simulink model "uwb_hw_cosim_kintex"  (Simulink 8.0)
settings: Solver=ode45  StartTime=0.0  StopTime=33  RelTol=1e-3
InitFcn:
  | clear
  | %set_channel;
  | load channel;
  | Int_Data_input;
StopFcn:
  | bit_to_dec_excel;
  | abc=1;
values from neighbouring files (symbols this model uses):
  bit_rate = 9.7656e5    (= 976560)    [Int_Data_input.m]
undefined symbols (not defined in the file or in its folder): rsgenpoly
libraries: commutil2 x88, simulink x53, dspmtrx3 x32, dspindex x16, commcnvcod2 x8, commblkcod2 x8, dspsigops x3, commsink2 x2, xbsIndex_r4 x1, commchan3 x1, JTAGRuntimeCosim_r4 x1
(part 4 of 5)

== system uwb_hw_cosim_kintex/Subsystem2/Transmit2/Spreading/Hop10/Subsystem5 ==
  In1 : Inport
  matrix : Inport  Port=2
  CONST3 : Constant  Value=zeros(1,320)  VectorParams1D=off  OutDataTypeStr=int8  SampleTime=1
      settings: SamplingMode=Frame based
  Compare To Zero : simulink/Logic and Bit Operations/Compare To Zero  relop=>  OutDataTypeStr=uint8  ZeroCross=off
  Enabled Subsystem : Subsystem  TreatAsAtomicUnit=on
  Enabled Subsystem1 : Subsystem  TreatAsAtomicUnit=on
  Logical Operator : Logic  Operator=NOT  AllPortsSameDT=off  OutDataTypeStr=boolean
  Merge : Merge
  Reshape2 : Reshape  OutputDimensionality=Column vector (2-D)  OutputDimensions=[10,1]
  Out1 : Outport
  wires:
  CONST3/1 -> Reshape2/1
  Logical Operator/1 -> Enabled Subsystem/Enable
  Enabled Subsystem/1(Out1) -> Merge/2
  Enabled Subsystem1/1(Out1) -> Merge/1
  Compare To Zero/1 -> Enabled Subsystem1/Enable, Logical Operator/1
  Reshape2/1 -> Enabled Subsystem1/1(In1)
  matrix/1 -> Enabled Subsystem/1(In1)
  In1/1 -> Compare To Zero/1
  Merge/1 -> Out1/1

== system uwb_hw_cosim_kintex/Subsystem2/Transmit2/Spreading/Hop11/Kron ==
  p : Inport
  -p : Inport  Port=2
  sel : Inport  Port=3
  Compare To Zero : simulink/Logic and Bit Operations/Compare To Zero  relop=>  OutDataTypeStr=uint8  ZeroCross=off
  Enabled Subsystem : Subsystem  TreatAsAtomicUnit=on
  Enabled Subsystem1 : Subsystem  TreatAsAtomicUnit=on
  Logical Operator : Logic  Operator=NOT  AllPortsSameDT=off  OutDataTypeStr=boolean
  Merge : Merge
  burst : Outport
  wires:
  Logical Operator/1 -> Enabled Subsystem/Enable
  Compare To Zero/1 -> Enabled Subsystem1/Enable, Logical Operator/1
  sel/1 -> Compare To Zero/1
  -p/1 -> Enabled Subsystem/1(In1)
  Enabled Subsystem/1(Out1) -> Merge/2
  Enabled Subsystem1/1(Out1) -> Merge/1
  p/1 -> Enabled Subsystem1/1(In1)
  Merge/1 -> burst/1

== system uwb_hw_cosim_kintex/Subsystem2/Transmit2/Spreading/Hop11/Kron1 ==
  p : Inport
  -p : Inport  Port=2
  sel : Inport  Port=3
  Compare To Zero : simulink/Logic and Bit Operations/Compare To Zero  relop=>  OutDataTypeStr=uint8  ZeroCross=off
  Enabled Subsystem : Subsystem  TreatAsAtomicUnit=on
  Enabled Subsystem1 : Subsystem  TreatAsAtomicUnit=on
  Logical Operator : Logic  Operator=NOT  AllPortsSameDT=off  OutDataTypeStr=boolean
  Merge : Merge
  burst : Outport
  wires:
  Merge/1 -> burst/1
  p/1 -> Enabled Subsystem1/1(In1)
  Enabled Subsystem1/1(Out1) -> Merge/1
  Enabled Subsystem/1(Out1) -> Merge/2
  -p/1 -> Enabled Subsystem/1(In1)
  sel/1 -> Compare To Zero/1
  Compare To Zero/1 -> Logical Operator/1, Enabled Subsystem1/Enable
  Logical Operator/1 -> Enabled Subsystem/Enable

== system uwb_hw_cosim_kintex/Subsystem2/Transmit2/Spreading/Hop11/Subsystem2 ==
  note: 16bit cua S mã hóa 1 cum xung gause 320 diem, them 7x320 diem 0
      | de tao ra 1/2 frame chua tin hieu
  In1 : Inport
  Buffer 48bit1 : Buffer  N=16
  Frame Conversion1 : FrameConversion
  Reshape3 : Reshape  OutputDimensionality=Customize  OutputDimensions=[320,1]
  Transpose1 : dspmtrx3/Transpose  Hermitian=off  overflowFlag=off
  Out1 : Outport
  wires:
  Frame Conversion1/1 -> Out1/1
  In1/1 -> Buffer 48bit1/1
  Reshape3/1 -> Frame Conversion1/1
  Transpose1/1 -> Reshape3/1
  Buffer 48bit1/1 -> Transpose1/1

== system uwb_hw_cosim_kintex/Subsystem2/Transmit2/Spreading/Hop11/Subsystem3 ==
  In1 : Inport
  Add1 : Sum  Inputs=+-
  Bi2De2 : commutil2/Bit to Integer Converter  nbits=2  bitOrder=MSB first  signedOutputValues=Unsigned  outDtype=int8  outDtypeSigned=Inherit via internal rule
  Gain2 : Gain  Gain=0.5  OutDataTypeStr=int8  RndMeth=Zero
  Gain4 : Gain  Gain=2  OutDataTypeStr=int8
  position : Outport
  sign : Outport  Port=2
  wires:
  Add1/1 -> position/1
  Bi2De2/1 -> Gain2/1, Add1/1
  Gain4/1 -> Add1/2
  Gain2/1 -> sign/1, Gain4/1
  In1/1 -> Bi2De2/1

== system uwb_hw_cosim_kintex/Subsystem2/Transmit2/Spreading/Hop11/Subsystem5 ==
  In1 : Inport
  matrix : Inport  Port=2
  CONST3 : Constant  Value=zeros(1,320)  VectorParams1D=off  OutDataTypeStr=int8  SampleTime=1
      settings: SamplingMode=Frame based
  Compare To Zero : simulink/Logic and Bit Operations/Compare To Zero  relop=>  OutDataTypeStr=uint8  ZeroCross=off
  Enabled Subsystem : Subsystem  TreatAsAtomicUnit=on
  Enabled Subsystem1 : Subsystem  TreatAsAtomicUnit=on
  Logical Operator : Logic  Operator=NOT  AllPortsSameDT=off  OutDataTypeStr=boolean
  Merge : Merge
  Reshape2 : Reshape  OutputDimensionality=Column vector (2-D)  OutputDimensions=[10,1]
  Out1 : Outport
  wires:
  Merge/1 -> Out1/1
  In1/1 -> Compare To Zero/1
  matrix/1 -> Enabled Subsystem/1(In1)
  Reshape2/1 -> Enabled Subsystem1/1(In1)
  Compare To Zero/1 -> Logical Operator/1, Enabled Subsystem1/Enable
  Enabled Subsystem1/1(Out1) -> Merge/1
  Enabled Subsystem/1(Out1) -> Merge/2
  Logical Operator/1 -> Enabled Subsystem/Enable
  CONST3/1 -> Reshape2/1

== system uwb_hw_cosim_kintex/Subsystem2/Transmit2/Spreading/Hop12/Kron ==
  p : Inport
  -p : Inport  Port=2
  sel : Inport  Port=3
  Compare To Zero : simulink/Logic and Bit Operations/Compare To Zero  relop=>  OutDataTypeStr=uint8  ZeroCross=off
  Enabled Subsystem : Subsystem  TreatAsAtomicUnit=on
  Enabled Subsystem1 : Subsystem  TreatAsAtomicUnit=on
  Logical Operator : Logic  Operator=NOT  AllPortsSameDT=off  OutDataTypeStr=boolean
  Merge : Merge
  burst : Outport
  wires:
  Logical Operator/1 -> Enabled Subsystem/Enable
  Compare To Zero/1 -> Enabled Subsystem1/Enable, Logical Operator/1
  sel/1 -> Compare To Zero/1
  -p/1 -> Enabled Subsystem/1(In1)
  Enabled Subsystem/1(Out1) -> Merge/2
  Enabled Subsystem1/1(Out1) -> Merge/1
  p/1 -> Enabled Subsystem1/1(In1)
  Merge/1 -> burst/1

== system uwb_hw_cosim_kintex/Subsystem2/Transmit2/Spreading/Hop12/Kron1 ==
  p : Inport
  -p : Inport  Port=2
  sel : Inport  Port=3
  Compare To Zero : simulink/Logic and Bit Operations/Compare To Zero  relop=>  OutDataTypeStr=uint8  ZeroCross=off
  Enabled Subsystem : Subsystem  TreatAsAtomicUnit=on
  Enabled Subsystem1 : Subsystem  TreatAsAtomicUnit=on
  Logical Operator : Logic  Operator=NOT  AllPortsSameDT=off  OutDataTypeStr=boolean
  Merge : Merge
  burst : Outport
  wires:
  Merge/1 -> burst/1
  p/1 -> Enabled Subsystem1/1(In1)
  Enabled Subsystem1/1(Out1) -> Merge/1
  Enabled Subsystem/1(Out1) -> Merge/2
  -p/1 -> Enabled Subsystem/1(In1)
  sel/1 -> Compare To Zero/1
  Compare To Zero/1 -> Logical Operator/1, Enabled Subsystem1/Enable
  Logical Operator/1 -> Enabled Subsystem/Enable

== system uwb_hw_cosim_kintex/Subsystem2/Transmit2/Spreading/Hop12/Subsystem2 ==
  note: 16bit cua S mã hóa 1 cum xung gause 320 diem, them 7x320 diem 0
      | de tao ra 1/2 frame chua tin hieu
  In1 : Inport
  Buffer 48bit1 : Buffer  N=16
  Frame Conversion1 : FrameConversion
  Reshape3 : Reshape  OutputDimensionality=Customize  OutputDimensions=[320,1]
  Transpose1 : dspmtrx3/Transpose  Hermitian=off  overflowFlag=off
  Out1 : Outport
  wires:
  Frame Conversion1/1 -> Out1/1
  In1/1 -> Buffer 48bit1/1
  Reshape3/1 -> Frame Conversion1/1
  Transpose1/1 -> Reshape3/1
  Buffer 48bit1/1 -> Transpose1/1

== system uwb_hw_cosim_kintex/Subsystem2/Transmit2/Spreading/Hop12/Subsystem3 ==
  In1 : Inport
  Add1 : Sum  Inputs=+-
  Bi2De2 : commutil2/Bit to Integer Converter  nbits=2  bitOrder=MSB first  signedOutputValues=Unsigned  outDtype=int8  outDtypeSigned=Inherit via internal rule
  Gain2 : Gain  Gain=0.5  OutDataTypeStr=int8  RndMeth=Zero
  Gain4 : Gain  Gain=2  OutDataTypeStr=int8
  position : Outport
  sign : Outport  Port=2
  wires:
  Add1/1 -> position/1
  Bi2De2/1 -> Gain2/1, Add1/1
  Gain4/1 -> Add1/2
  Gain2/1 -> sign/1, Gain4/1
  In1/1 -> Bi2De2/1

== system uwb_hw_cosim_kintex/Subsystem2/Transmit2/Spreading/Hop12/Subsystem5 ==
  In1 : Inport
  matrix : Inport  Port=2
  CONST3 : Constant  Value=zeros(1,320)  VectorParams1D=off  OutDataTypeStr=int8  SampleTime=1
      settings: SamplingMode=Frame based
  Compare To Zero : simulink/Logic and Bit Operations/Compare To Zero  relop===  OutDataTypeStr=uint8  ZeroCross=off
  Enabled Subsystem : Subsystem  TreatAsAtomicUnit=on
  Enabled Subsystem1 : Subsystem  TreatAsAtomicUnit=on
  Logical Operator : Logic  Operator=NOT  AllPortsSameDT=off  OutDataTypeStr=boolean
  Merge : Merge
  Reshape2 : Reshape  OutputDimensionality=Column vector (2-D)  OutputDimensions=[10,1]
  Out1 : Outport
  wires:
  Merge/1 -> Out1/1
  In1/1 -> Compare To Zero/1
  Reshape2/1 -> Enabled Subsystem1/1(In1)
  Compare To Zero/1 -> Logical Operator/1, Enabled Subsystem1/Enable
  Enabled Subsystem1/1(Out1) -> Merge/1
  Enabled Subsystem/1(Out1) -> Merge/2
  Logical Operator/1 -> Enabled Subsystem/Enable
  CONST3/1 -> Reshape2/1
  matrix/1 -> Enabled Subsystem/1(In1)

== system uwb_hw_cosim_kintex/Subsystem2/Transmit2/Spreading/Hop13/Kron ==
  p : Inport
  -p : Inport  Port=2
  sel : Inport  Port=3
  Compare To Zero : simulink/Logic and Bit Operations/Compare To Zero  relop=>  OutDataTypeStr=uint8  ZeroCross=off
  Enabled Subsystem : Subsystem  TreatAsAtomicUnit=on
  Enabled Subsystem1 : Subsystem  TreatAsAtomicUnit=on
  Logical Operator : Logic  Operator=NOT  AllPortsSameDT=off  OutDataTypeStr=boolean
  Merge : Merge
  burst : Outport
  wires:
  Merge/1 -> burst/1
  p/1 -> Enabled Subsystem1/1(In1)
  Enabled Subsystem1/1(Out1) -> Merge/1
  Enabled Subsystem/1(Out1) -> Merge/2
  -p/1 -> Enabled Subsystem/1(In1)
  sel/1 -> Compare To Zero/1
  Compare To Zero/1 -> Logical Operator/1, Enabled Subsystem1/Enable
  Logical Operator/1 -> Enabled Subsystem/Enable

== system uwb_hw_cosim_kintex/Subsystem2/Transmit2/Spreading/Hop13/Kron1 ==
  p : Inport
  -p : Inport  Port=2
  sel : Inport  Port=3
  Compare To Zero : simulink/Logic and Bit Operations/Compare To Zero  relop=>  OutDataTypeStr=uint8  ZeroCross=off
  Enabled Subsystem : Subsystem  TreatAsAtomicUnit=on
  Enabled Subsystem1 : Subsystem  TreatAsAtomicUnit=on
  Logical Operator : Logic  Operator=NOT  AllPortsSameDT=off  OutDataTypeStr=boolean
  Merge : Merge
  burst : Outport
  wires:
  Logical Operator/1 -> Enabled Subsystem/Enable
  Compare To Zero/1 -> Enabled Subsystem1/Enable, Logical Operator/1
  sel/1 -> Compare To Zero/1
  -p/1 -> Enabled Subsystem/1(In1)
  Enabled Subsystem/1(Out1) -> Merge/2
  Enabled Subsystem1/1(Out1) -> Merge/1
  p/1 -> Enabled Subsystem1/1(In1)
  Merge/1 -> burst/1

== system uwb_hw_cosim_kintex/Subsystem2/Transmit2/Spreading/Hop13/Subsystem2 ==
  note: 16bit cua S mã hóa 1 cum xung gause 320 diem, them 7x320 diem 0
      | de tao ra 1/2 frame chua tin hieu
  In1 : Inport
  Buffer 48bit1 : Buffer  N=16
  Frame Conversion1 : FrameConversion
  Reshape3 : Reshape  OutputDimensionality=Customize  OutputDimensions=[320,1]
  Transpose1 : dspmtrx3/Transpose  Hermitian=off  overflowFlag=off
  Out1 : Outport
  wires:
  Buffer 48bit1/1 -> Transpose1/1
  Transpose1/1 -> Reshape3/1
  Reshape3/1 -> Frame Conversion1/1
  In1/1 -> Buffer 48bit1/1
  Frame Conversion1/1 -> Out1/1

== system uwb_hw_cosim_kintex/Subsystem2/Transmit2/Spreading/Hop13/Subsystem3 ==
  In1 : Inport
  Add1 : Sum  Inputs=+-
  Bi2De2 : commutil2/Bit to Integer Converter  nbits=2  bitOrder=MSB first  signedOutputValues=Unsigned  outDtype=int8  outDtypeSigned=Inherit via internal rule
  Gain2 : Gain  Gain=0.5  OutDataTypeStr=int8  RndMeth=Zero
  Gain4 : Gain  Gain=2  OutDataTypeStr=int8
  position : Outport
  sign : Outport  Port=2
  wires:
  In1/1 -> Bi2De2/1
  Gain2/1 -> Gain4/1, sign/1
  Gain4/1 -> Add1/2
  Bi2De2/1 -> Add1/1, Gain2/1
  Add1/1 -> position/1

== system uwb_hw_cosim_kintex/Subsystem2/Transmit2/Spreading/Hop13/Subsystem5 ==
  In1 : Inport
  matrix : Inport  Port=2
  CONST3 : Constant  Value=zeros(1,320)  VectorParams1D=off  OutDataTypeStr=int8  SampleTime=1
      settings: SamplingMode=Frame based
  Compare To Zero : simulink/Logic and Bit Operations/Compare To Zero  relop===  OutDataTypeStr=uint8  ZeroCross=off
  Enabled Subsystem : Subsystem  TreatAsAtomicUnit=on
  Enabled Subsystem1 : Subsystem  TreatAsAtomicUnit=on
  Logical Operator : Logic  Operator=NOT  AllPortsSameDT=off  OutDataTypeStr=boolean
  Merge : Merge
  Reshape2 : Reshape  OutputDimensionality=Column vector (2-D)  OutputDimensions=[10,1]
  Out1 : Outport
  wires:
  matrix/1 -> Enabled Subsystem/1(In1)
  CONST3/1 -> Reshape2/1
  Logical Operator/1 -> Enabled Subsystem/Enable
  Enabled Subsystem/1(Out1) -> Merge/2
  Enabled Subsystem1/1(Out1) -> Merge/1
  Compare To Zero/1 -> Enabled Subsystem1/Enable, Logical Operator/1
  Reshape2/1 -> Enabled Subsystem1/1(In1)
  In1/1 -> Compare To Zero/1
  Merge/1 -> Out1/1

== system uwb_hw_cosim_kintex/Subsystem2/Transmit2/Spreading/Hop14/Kron ==
  p : Inport
  -p : Inport  Port=2
  sel : Inport  Port=3
  Compare To Zero : simulink/Logic and Bit Operations/Compare To Zero  relop=>  OutDataTypeStr=uint8  ZeroCross=off
  Enabled Subsystem : Subsystem  TreatAsAtomicUnit=on
  Enabled Subsystem1 : Subsystem  TreatAsAtomicUnit=on
  Logical Operator : Logic  Operator=NOT  AllPortsSameDT=off  OutDataTypeStr=boolean
  Merge : Merge
  burst : Outport
  wires:
  Logical Operator/1 -> Enabled Subsystem/Enable
  Compare To Zero/1 -> Enabled Subsystem1/Enable, Logical Operator/1
  sel/1 -> Compare To Zero/1
  -p/1 -> Enabled Subsystem/1(In1)
  Enabled Subsystem/1(Out1) -> Merge/2
  Enabled Subsystem1/1(Out1) -> Merge/1
  p/1 -> Enabled Subsystem1/1(In1)
  Merge/1 -> burst/1

== system uwb_hw_cosim_kintex/Subsystem2/Transmit2/Spreading/Hop14/Kron1 ==
  p : Inport
  -p : Inport  Port=2
  sel : Inport  Port=3
  Compare To Zero : simulink/Logic and Bit Operations/Compare To Zero  relop=>  OutDataTypeStr=uint8  ZeroCross=off
  Enabled Subsystem : Subsystem  TreatAsAtomicUnit=on
  Enabled Subsystem1 : Subsystem  TreatAsAtomicUnit=on
  Logical Operator : Logic  Operator=NOT  AllPortsSameDT=off  OutDataTypeStr=boolean
  Merge : Merge
  burst : Outport
  wires:
  Merge/1 -> burst/1
  p/1 -> Enabled Subsystem1/1(In1)
  Enabled Subsystem1/1(Out1) -> Merge/1
  Enabled Subsystem/1(Out1) -> Merge/2
  -p/1 -> Enabled Subsystem/1(In1)
  sel/1 -> Compare To Zero/1
  Compare To Zero/1 -> Logical Operator/1, Enabled Subsystem1/Enable
  Logical Operator/1 -> Enabled Subsystem/Enable

== system uwb_hw_cosim_kintex/Subsystem2/Transmit2/Spreading/Hop14/Subsystem2 ==
  note: 16bit cua S mã hóa 1 cum xung gause 320 diem, them 7x320 diem 0
      | de tao ra 1/2 frame chua tin hieu
  In1 : Inport
  Buffer 48bit1 : Buffer  N=16
  Frame Conversion1 : FrameConversion
  Reshape3 : Reshape  OutputDimensionality=Customize  OutputDimensions=[320,1]
  Transpose1 : dspmtrx3/Transpose  Hermitian=off  overflowFlag=off
  Out1 : Outport
  wires:
  Frame Conversion1/1 -> Out1/1
  In1/1 -> Buffer 48bit1/1
  Reshape3/1 -> Frame Conversion1/1
  Transpose1/1 -> Reshape3/1
  Buffer 48bit1/1 -> Transpose1/1

== system uwb_hw_cosim_kintex/Subsystem2/Transmit2/Spreading/Hop14/Subsystem3 ==
  In1 : Inport
  Add1 : Sum  Inputs=+-
  Bi2De2 : commutil2/Bit to Integer Converter  nbits=2  bitOrder=MSB first  signedOutputValues=Unsigned  outDtype=int8  outDtypeSigned=Inherit via internal rule
  Gain2 : Gain  Gain=0.5  OutDataTypeStr=int8  RndMeth=Zero
  Gain4 : Gain  Gain=2  OutDataTypeStr=int8
  position : Outport
  sign : Outport  Port=2
  wires:
  Add1/1 -> position/1
  Bi2De2/1 -> Gain2/1, Add1/1
  Gain4/1 -> Add1/2
  Gain2/1 -> sign/1, Gain4/1
  In1/1 -> Bi2De2/1

== system uwb_hw_cosim_kintex/Subsystem2/Transmit2/Spreading/Hop14/Subsystem5 ==
  In1 : Inport
  matrix : Inport  Port=2
  CONST3 : Constant  Value=zeros(1,320)  VectorParams1D=off  OutDataTypeStr=int8  SampleTime=1
      settings: SamplingMode=Frame based
  Compare To Zero : simulink/Logic and Bit Operations/Compare To Zero  relop===  OutDataTypeStr=uint8  ZeroCross=off
  Enabled Subsystem : Subsystem  TreatAsAtomicUnit=on
  Enabled Subsystem1 : Subsystem  TreatAsAtomicUnit=on
  Logical Operator : Logic  Operator=NOT  AllPortsSameDT=off  OutDataTypeStr=boolean
  Merge : Merge
  Reshape2 : Reshape  OutputDimensionality=Column vector (2-D)  OutputDimensions=[10,1]
  Out1 : Outport
  wires:
  Merge/1 -> Out1/1
  In1/1 -> Compare To Zero/1
  Reshape2/1 -> Enabled Subsystem1/1(In1)
  Compare To Zero/1 -> Logical Operator/1, Enabled Subsystem1/Enable
  Enabled Subsystem1/1(Out1) -> Merge/1
  Enabled Subsystem/1(Out1) -> Merge/2
  Logical Operator/1 -> Enabled Subsystem/Enable
  CONST3/1 -> Reshape2/1
  matrix/1 -> Enabled Subsystem/1(In1)

== system uwb_hw_cosim_kintex/Subsystem2/Transmit2/Spreading/Hop15/Kron ==
  p : Inport
  -p : Inport  Port=2
  sel : Inport  Port=3
  Compare To Zero : simulink/Logic and Bit Operations/Compare To Zero  relop=>  OutDataTypeStr=uint8  ZeroCross=off
  Enabled Subsystem : Subsystem  TreatAsAtomicUnit=on
  Enabled Subsystem1 : Subsystem  TreatAsAtomicUnit=on
  Logical Operator : Logic  Operator=NOT  AllPortsSameDT=off  OutDataTypeStr=boolean
  Merge : Merge
  burst : Outport
  wires:
  Merge/1 -> burst/1
  p/1 -> Enabled Subsystem1/1(In1)
  Enabled Subsystem1/1(Out1) -> Merge/1
  Enabled Subsystem/1(Out1) -> Merge/2
  -p/1 -> Enabled Subsystem/1(In1)
  sel/1 -> Compare To Zero/1
  Compare To Zero/1 -> Logical Operator/1, Enabled Subsystem1/Enable
  Logical Operator/1 -> Enabled Subsystem/Enable

== system uwb_hw_cosim_kintex/Subsystem2/Transmit2/Spreading/Hop15/Kron1 ==
  p : Inport
  -p : Inport  Port=2
  sel : Inport  Port=3
  Compare To Zero : simulink/Logic and Bit Operations/Compare To Zero  relop=>  OutDataTypeStr=uint8  ZeroCross=off
  Enabled Subsystem : Subsystem  TreatAsAtomicUnit=on
  Enabled Subsystem1 : Subsystem  TreatAsAtomicUnit=on
  Logical Operator : Logic  Operator=NOT  AllPortsSameDT=off  OutDataTypeStr=boolean
  Merge : Merge
  burst : Outport
  wires:
  Logical Operator/1 -> Enabled Subsystem/Enable
  Compare To Zero/1 -> Enabled Subsystem1/Enable, Logical Operator/1
  sel/1 -> Compare To Zero/1
  -p/1 -> Enabled Subsystem/1(In1)
  Enabled Subsystem/1(Out1) -> Merge/2
  Enabled Subsystem1/1(Out1) -> Merge/1
  p/1 -> Enabled Subsystem1/1(In1)
  Merge/1 -> burst/1

== system uwb_hw_cosim_kintex/Subsystem2/Transmit2/Spreading/Hop15/Subsystem2 ==
  note: 16bit cua S mã hóa 1 cum xung gause 320 diem, them 7x320 diem 0
      | de tao ra 1/2 frame chua tin hieu
  In1 : Inport
  Buffer 48bit1 : Buffer  N=16
  Frame Conversion1 : FrameConversion
  Reshape3 : Reshape  OutputDimensionality=Customize  OutputDimensions=[320,1]
  Transpose1 : dspmtrx3/Transpose  Hermitian=off  overflowFlag=off
  Out1 : Outport
  wires:
  Buffer 48bit1/1 -> Transpose1/1
  Transpose1/1 -> Reshape3/1
  Reshape3/1 -> Frame Conversion1/1
  In1/1 -> Buffer 48bit1/1
  Frame Conversion1/1 -> Out1/1

== system uwb_hw_cosim_kintex/Subsystem2/Transmit2/Spreading/Hop15/Subsystem3 ==
  In1 : Inport
  Add1 : Sum  Inputs=+-
  Bi2De2 : commutil2/Bit to Integer Converter  nbits=2  bitOrder=MSB first  signedOutputValues=Unsigned  outDtype=int8  outDtypeSigned=Inherit via internal rule
  Gain2 : Gain  Gain=0.5  OutDataTypeStr=int8  RndMeth=Zero
  Gain4 : Gain  Gain=2  OutDataTypeStr=int8
  position : Outport
  sign : Outport  Port=2
  wires:
  In1/1 -> Bi2De2/1
  Gain2/1 -> Gain4/1, sign/1
  Gain4/1 -> Add1/2
  Bi2De2/1 -> Add1/1, Gain2/1
  Add1/1 -> position/1

== system uwb_hw_cosim_kintex/Subsystem2/Transmit2/Spreading/Hop15/Subsystem5 ==
  In1 : Inport
  matrix : Inport  Port=2
  CONST3 : Constant  Value=zeros(1,320)  VectorParams1D=off  OutDataTypeStr=int8  SampleTime=1
      settings: SamplingMode=Frame based
  Compare To Zero : simulink/Logic and Bit Operations/Compare To Zero  relop===  OutDataTypeStr=uint8  ZeroCross=off
  Enabled Subsystem : Subsystem  TreatAsAtomicUnit=on
  Enabled Subsystem1 : Subsystem  TreatAsAtomicUnit=on
  Logical Operator : Logic  Operator=NOT  AllPortsSameDT=off  OutDataTypeStr=boolean
  Merge : Merge
  Reshape2 : Reshape  OutputDimensionality=Column vector (2-D)  OutputDimensions=[10,1]
  Out1 : Outport
  wires:
  matrix/1 -> Enabled Subsystem/1(In1)
  CONST3/1 -> Reshape2/1
  Logical Operator/1 -> Enabled Subsystem/Enable
  Enabled Subsystem/1(Out1) -> Merge/2
  Enabled Subsystem1/1(Out1) -> Merge/1
  Compare To Zero/1 -> Enabled Subsystem1/Enable, Logical Operator/1
  Reshape2/1 -> Enabled Subsystem1/1(In1)
  In1/1 -> Compare To Zero/1
  Merge/1 -> Out1/1

== system uwb_hw_cosim_kintex/Subsystem2/Transmit2/Spreading/Hop17/Kron ==
  p : Inport
  -p : Inport  Port=2
  sel : Inport  Port=3
  Compare To Zero : simulink/Logic and Bit Operations/Compare To Zero  relop=>  OutDataTypeStr=uint8  ZeroCross=off
  Enabled Subsystem : Subsystem  TreatAsAtomicUnit=on
  Enabled Subsystem1 : Subsystem  TreatAsAtomicUnit=on
  Logical Operator : Logic  Operator=NOT  AllPortsSameDT=off  OutDataTypeStr=boolean
  Merge : Merge
  burst : Outport
  wires:
  Merge/1 -> burst/1
  p/1 -> Enabled Subsystem1/1(In1)
  Enabled Subsystem1/1(Out1) -> Merge/1
  Enabled Subsystem/1(Out1) -> Merge/2
  -p/1 -> Enabled Subsystem/1(In1)
  sel/1 -> Compare To Zero/1
  Compare To Zero/1 -> Logical Operator/1, Enabled Subsystem1/Enable
  Logical Operator/1 -> Enabled Subsystem/Enable

== system uwb_hw_cosim_kintex/Subsystem2/Transmit2/Spreading/Hop17/Kron1 ==
  p : Inport
  -p : Inport  Port=2
  sel : Inport  Port=3
  Compare To Zero : simulink/Logic and Bit Operations/Compare To Zero  relop=>  OutDataTypeStr=uint8  ZeroCross=off
  Enabled Subsystem : Subsystem  TreatAsAtomicUnit=on
  Enabled Subsystem1 : Subsystem  TreatAsAtomicUnit=on
  Logical Operator : Logic  Operator=NOT  AllPortsSameDT=off  OutDataTypeStr=boolean
  Merge : Merge
  burst : Outport
  wires:
  Logical Operator/1 -> Enabled Subsystem/Enable
  Compare To Zero/1 -> Enabled Subsystem1/Enable, Logical Operator/1
  sel/1 -> Compare To Zero/1
  -p/1 -> Enabled Subsystem/1(In1)
  Enabled Subsystem/1(Out1) -> Merge/2
  Enabled Subsystem1/1(Out1) -> Merge/1
  p/1 -> Enabled Subsystem1/1(In1)
  Merge/1 -> burst/1

== system uwb_hw_cosim_kintex/Subsystem2/Transmit2/Spreading/Hop17/Subsystem2 ==
  note: 16bit cua S mã hóa 1 cum xung gause 320 diem, them 7x320 diem 0
      | de tao ra 1/2 frame chua tin hieu
  In1 : Inport
  Buffer 48bit1 : Buffer  N=16
  Frame Conversion1 : FrameConversion
  Reshape3 : Reshape  OutputDimensionality=Customize  OutputDimensions=[320,1]
  Transpose1 : dspmtrx3/Transpose  Hermitian=off  overflowFlag=off
  Out1 : Outport
  wires:
  Buffer 48bit1/1 -> Transpose1/1
  Transpose1/1 -> Reshape3/1
  Reshape3/1 -> Frame Conversion1/1
  In1/1 -> Buffer 48bit1/1
  Frame Conversion1/1 -> Out1/1

== system uwb_hw_cosim_kintex/Subsystem2/Transmit2/Spreading/Hop17/Subsystem3 ==
  In1 : Inport
  Add1 : Sum  Inputs=+-
  Bi2De2 : commutil2/Bit to Integer Converter  nbits=2  bitOrder=MSB first  signedOutputValues=Unsigned  outDtype=int8  outDtypeSigned=Inherit via internal rule
  Gain2 : Gain  Gain=0.5  OutDataTypeStr=int8  RndMeth=Zero
  Gain4 : Gain  Gain=2  OutDataTypeStr=int8
  position : Outport
  sign : Outport  Port=2
  wires:
  In1/1 -> Bi2De2/1
  Gain2/1 -> Gain4/1, sign/1
  Gain4/1 -> Add1/2
  Bi2De2/1 -> Add1/1, Gain2/1
  Add1/1 -> position/1

== system uwb_hw_cosim_kintex/Subsystem2/Transmit2/Spreading/Hop17/Subsystem5 ==
  In1 : Inport
  matrix : Inport  Port=2
  CONST3 : Constant  Value=zeros(1,320)  VectorParams1D=off  OutDataTypeStr=int8  SampleTime=1
      settings: SamplingMode=Frame based
  Compare To Zero : simulink/Logic and Bit Operations/Compare To Zero  relop===  OutDataTypeStr=uint8  ZeroCross=off
  Enabled Subsystem : Subsystem  TreatAsAtomicUnit=on
  Enabled Subsystem1 : Subsystem  TreatAsAtomicUnit=on
  Logical Operator : Logic  Operator=NOT  AllPortsSameDT=off  OutDataTypeStr=boolean
  Merge : Merge
  Reshape2 : Reshape  OutputDimensionality=Column vector (2-D)  OutputDimensions=[10,1]
  Out1 : Outport
  wires:
  matrix/1 -> Enabled Subsystem/1(In1)
  CONST3/1 -> Reshape2/1
  Logical Operator/1 -> Enabled Subsystem/Enable
  Enabled Subsystem/1(Out1) -> Merge/2
  Enabled Subsystem1/1(Out1) -> Merge/1
  Compare To Zero/1 -> Enabled Subsystem1/Enable, Logical Operator/1
  Reshape2/1 -> Enabled Subsystem1/1(In1)
  In1/1 -> Compare To Zero/1
  Merge/1 -> Out1/1

== system uwb_hw_cosim_kintex/Subsystem2/Transmit2/Spreading/Hop2/Kron ==
  p : Inport
  -p : Inport  Port=2
  sel : Inport  Port=3
  Compare To Zero : simulink/Logic and Bit Operations/Compare To Zero  relop=>  OutDataTypeStr=uint8  ZeroCross=off
  Enabled Subsystem : Subsystem  TreatAsAtomicUnit=on
  Enabled Subsystem1 : Subsystem  TreatAsAtomicUnit=on
  Logical Operator : Logic  Operator=NOT  AllPortsSameDT=off  OutDataTypeStr=boolean
  Merge : Merge
  burst : Outport
  wires:
  Merge/1 -> burst/1
  p/1 -> Enabled Subsystem1/1(In1)
  Enabled Subsystem1/1(Out1) -> Merge/1
  Enabled Subsystem/1(Out1) -> Merge/2
  -p/1 -> Enabled Subsystem/1(In1)
  sel/1 -> Compare To Zero/1
  Compare To Zero/1 -> Logical Operator/1, Enabled Subsystem1/Enable
  Logical Operator/1 -> Enabled Subsystem/Enable

== system uwb_hw_cosim_kintex/Subsystem2/Transmit2/Spreading/Hop2/Kron1 ==
  p : Inport
  -p : Inport  Port=2
  sel : Inport  Port=3
  Compare To Zero : simulink/Logic and Bit Operations/Compare To Zero  relop=>  OutDataTypeStr=uint8  ZeroCross=off
  Enabled Subsystem : Subsystem  TreatAsAtomicUnit=on
  Enabled Subsystem1 : Subsystem  TreatAsAtomicUnit=on
  Logical Operator : Logic  Operator=NOT  AllPortsSameDT=off  OutDataTypeStr=boolean
  Merge : Merge
  burst : Outport
  wires:
  Logical Operator/1 -> Enabled Subsystem/Enable
  Compare To Zero/1 -> Enabled Subsystem1/Enable, Logical Operator/1
  sel/1 -> Compare To Zero/1
  -p/1 -> Enabled Subsystem/1(In1)
  Enabled Subsystem/1(Out1) -> Merge/2
  Enabled Subsystem1/1(Out1) -> Merge/1
  p/1 -> Enabled Subsystem1/1(In1)
  Merge/1 -> burst/1

== system uwb_hw_cosim_kintex/Subsystem2/Transmit2/Spreading/Hop2/Subsystem2 ==
  note: 16bit cua S mã hóa 1 cum xung gause 320 diem, them 7x320 diem 0
      | de tao ra 1/2 frame chua tin hieu
  In1 : Inport
  Buffer 48bit1 : Buffer  N=16
  Frame Conversion1 : FrameConversion
  Reshape3 : Reshape  OutputDimensionality=Customize  OutputDimensions=[320,1]
  Transpose1 : dspmtrx3/Transpose  Hermitian=off  overflowFlag=off
  Out1 : Outport
  wires:
  Buffer 48bit1/1 -> Transpose1/1
  Transpose1/1 -> Reshape3/1
  Reshape3/1 -> Frame Conversion1/1
  In1/1 -> Buffer 48bit1/1
  Frame Conversion1/1 -> Out1/1

== system uwb_hw_cosim_kintex/Subsystem2/Transmit2/Spreading/Hop2/Subsystem3 ==
  In1 : Inport
  Add1 : Sum  Inputs=+-
  Bi2De2 : commutil2/Bit to Integer Converter  nbits=2  bitOrder=MSB first  signedOutputValues=Unsigned  outDtype=int8  outDtypeSigned=Inherit via internal rule
  Gain2 : Gain  Gain=0.5  OutDataTypeStr=int8  RndMeth=Zero
  Gain4 : Gain  Gain=2  OutDataTypeStr=int8
  position : Outport
  sign : Outport  Port=2
  wires:
  In1/1 -> Bi2De2/1
  Gain2/1 -> Gain4/1, sign/1
  Gain4/1 -> Add1/2
  Bi2De2/1 -> Add1/1, Gain2/1
  Add1/1 -> position/1

== system uwb_hw_cosim_kintex/Subsystem2/Transmit2/Spreading/Hop2/Subsystem5 ==
  In1 : Inport
  matrix : Inport  Port=2
  CONST3 : Constant  Value=zeros(1,320)  VectorParams1D=off  OutDataTypeStr=int8  SampleTime=1
      settings: SamplingMode=Frame based
  Compare To Zero : simulink/Logic and Bit Operations/Compare To Zero  relop=>  OutDataTypeStr=uint8  ZeroCross=off
  Enabled Subsystem : Subsystem  TreatAsAtomicUnit=on
  Enabled Subsystem1 : Subsystem  TreatAsAtomicUnit=on
  Logical Operator : Logic  Operator=NOT  AllPortsSameDT=off  OutDataTypeStr=boolean
  Merge : Merge
  Reshape2 : Reshape  OutputDimensionality=Column vector (2-D)  OutputDimensions=[10,1]
  Out1 : Outport
  wires:
  CONST3/1 -> Reshape2/1
  Logical Operator/1 -> Enabled Subsystem/Enable
  Enabled Subsystem/1(Out1) -> Merge/2
  Enabled Subsystem1/1(Out1) -> Merge/1
  Compare To Zero/1 -> Enabled Subsystem1/Enable, Logical Operator/1
  Reshape2/1 -> Enabled Subsystem1/1(In1)
  matrix/1 -> Enabled Subsystem/1(In1)
  In1/1 -> Compare To Zero/1
  Merge/1 -> Out1/1

== system uwb_hw_cosim_kintex/Subsystem2/Transmit2/Spreading/Hop3/Kron ==
  p : Inport
  -p : Inport  Port=2
  sel : Inport  Port=3
  Compare To Zero : simulink/Logic and Bit Operations/Compare To Zero  relop=>  OutDataTypeStr=uint8  ZeroCross=off
  Enabled Subsystem : Subsystem  TreatAsAtomicUnit=on
  Enabled Subsystem1 : Subsystem  TreatAsAtomicUnit=on
  Logical Operator : Logic  Operator=NOT  AllPortsSameDT=off  OutDataTypeStr=boolean
  Merge : Merge
  burst : Outport
  wires:
  Logical Operator/1 -> Enabled Subsystem/Enable
  Compare To Zero/1 -> Enabled Subsystem1/Enable, Logical Operator/1
  sel/1 -> Compare To Zero/1
  -p/1 -> Enabled Subsystem/1(In1)
  Enabled Subsystem/1(Out1) -> Merge/2
  Enabled Subsystem1/1(Out1) -> Merge/1
  p/1 -> Enabled Subsystem1/1(In1)
  Merge/1 -> burst/1

== system uwb_hw_cosim_kintex/Subsystem2/Transmit2/Spreading/Hop3/Kron1 ==
  p : Inport
  -p : Inport  Port=2
  sel : Inport  Port=3
  Compare To Zero : simulink/Logic and Bit Operations/Compare To Zero  relop=>  OutDataTypeStr=uint8  ZeroCross=off
  Enabled Subsystem : Subsystem  TreatAsAtomicUnit=on
  Enabled Subsystem1 : Subsystem  TreatAsAtomicUnit=on
  Logical Operator : Logic  Operator=NOT  AllPortsSameDT=off  OutDataTypeStr=boolean
  Merge : Merge
  burst : Outport
  wires:
  Merge/1 -> burst/1
  p/1 -> Enabled Subsystem1/1(In1)
  Enabled Subsystem1/1(Out1) -> Merge/1
  Enabled Subsystem/1(Out1) -> Merge/2
  -p/1 -> Enabled Subsystem/1(In1)
  sel/1 -> Compare To Zero/1
  Compare To Zero/1 -> Logical Operator/1, Enabled Subsystem1/Enable
  Logical Operator/1 -> Enabled Subsystem/Enable

== system uwb_hw_cosim_kintex/Subsystem2/Transmit2/Spreading/Hop3/Subsystem2 ==
  note: 16bit cua S mã hóa 1 cum xung gause 320 diem, them 7x320 diem 0
      | de tao ra 1/2 frame chua tin hieu
  In1 : Inport
  Buffer 48bit1 : Buffer  N=16
  Frame Conversion1 : FrameConversion
  Reshape3 : Reshape  OutputDimensionality=Customize  OutputDimensions=[320,1]
  Transpose1 : dspmtrx3/Transpose  Hermitian=off  overflowFlag=off
  Out1 : Outport
  wires:
  Frame Conversion1/1 -> Out1/1
  In1/1 -> Buffer 48bit1/1
  Reshape3/1 -> Frame Conversion1/1
  Transpose1/1 -> Reshape3/1
  Buffer 48bit1/1 -> Transpose1/1

== system uwb_hw_cosim_kintex/Subsystem2/Transmit2/Spreading/Hop3/Subsystem3 ==
  In1 : Inport
  Add1 : Sum  Inputs=+-
  Bi2De2 : commutil2/Bit to Integer Converter  nbits=2  bitOrder=MSB first  signedOutputValues=Unsigned  outDtype=int8  outDtypeSigned=Inherit via internal rule
  Gain2 : Gain  Gain=0.5  OutDataTypeStr=int8  RndMeth=Zero
  Gain4 : Gain  Gain=2  OutDataTypeStr=int8
  position : Outport
  sign : Outport  Port=2
  wires:
  Add1/1 -> position/1
  Bi2De2/1 -> Gain2/1, Add1/1
  Gain4/1 -> Add1/2
  Gain2/1 -> sign/1, Gain4/1
  In1/1 -> Bi2De2/1

== system uwb_hw_cosim_kintex/Subsystem2/Transmit2/Spreading/Hop3/Subsystem5 ==
  In1 : Inport
  matrix : Inport  Port=2
  CONST3 : Constant  Value=zeros(1,320)  VectorParams1D=off  OutDataTypeStr=int8  SampleTime=1
      settings: SamplingMode=Frame based
  Compare To Zero : simulink/Logic and Bit Operations/Compare To Zero  relop=>  OutDataTypeStr=uint8  ZeroCross=off
  Enabled Subsystem : Subsystem  TreatAsAtomicUnit=on
  Enabled Subsystem1 : Subsystem  TreatAsAtomicUnit=on
  Logical Operator : Logic  Operator=NOT  AllPortsSameDT=off  OutDataTypeStr=boolean
  Merge : Merge
  Reshape2 : Reshape  OutputDimensionality=Column vector (2-D)  OutputDimensions=[10,1]
  Out1 : Outport
  wires:
  Merge/1 -> Out1/1
  In1/1 -> Compare To Zero/1
  matrix/1 -> Enabled Subsystem/1(In1)
  Reshape2/1 -> Enabled Subsystem1/1(In1)
  Compare To Zero/1 -> Logical Operator/1, Enabled Subsystem1/Enable
  Enabled Subsystem1/1(Out1) -> Merge/1
  Enabled Subsystem/1(Out1) -> Merge/2
  Logical Operator/1 -> Enabled Subsystem/Enable
  CONST3/1 -> Reshape2/1

== system uwb_hw_cosim_kintex/Subsystem2/Transmit2/Spreading/Hop4/Kron ==
  p : Inport
  -p : Inport  Port=2
  sel : Inport  Port=3
  Compare To Zero : simulink/Logic and Bit Operations/Compare To Zero  relop=>  OutDataTypeStr=uint8  ZeroCross=off
  Enabled Subsystem : Subsystem  TreatAsAtomicUnit=on
  Enabled Subsystem1 : Subsystem  TreatAsAtomicUnit=on
  Logical Operator : Logic  Operator=NOT  AllPortsSameDT=off  OutDataTypeStr=boolean
  Merge : Merge
  burst : Outport
  wires:
  Merge/1 -> burst/1
  p/1 -> Enabled Subsystem1/1(In1)
  Enabled Subsystem1/1(Out1) -> Merge/1
  Enabled Subsystem/1(Out1) -> Merge/2
  -p/1 -> Enabled Subsystem/1(In1)
  sel/1 -> Compare To Zero/1
  Compare To Zero/1 -> Logical Operator/1, Enabled Subsystem1/Enable
  Logical Operator/1 -> Enabled Subsystem/Enable

== system uwb_hw_cosim_kintex/Subsystem2/Transmit2/Spreading/Hop4/Kron1 ==
  p : Inport
  -p : Inport  Port=2
  sel : Inport  Port=3
  Compare To Zero : simulink/Logic and Bit Operations/Compare To Zero  relop=>  OutDataTypeStr=uint8  ZeroCross=off
  Enabled Subsystem : Subsystem  TreatAsAtomicUnit=on
  Enabled Subsystem1 : Subsystem  TreatAsAtomicUnit=on
  Logical Operator : Logic  Operator=NOT  AllPortsSameDT=off  OutDataTypeStr=boolean
  Merge : Merge
  burst : Outport
  wires:
  Logical Operator/1 -> Enabled Subsystem/Enable
  Compare To Zero/1 -> Enabled Subsystem1/Enable, Logical Operator/1
  sel/1 -> Compare To Zero/1
  -p/1 -> Enabled Subsystem/1(In1)
  Enabled Subsystem/1(Out1) -> Merge/2
  Enabled Subsystem1/1(Out1) -> Merge/1
  p/1 -> Enabled Subsystem1/1(In1)
  Merge/1 -> burst/1

== system uwb_hw_cosim_kintex/Subsystem2/Transmit2/Spreading/Hop4/Subsystem2 ==
  note: 16bit cua S mã hóa 1 cum xung gause 320 diem, them 7x320 diem 0
      | de tao ra 1/2 frame chua tin hieu
  In1 : Inport
  Buffer 48bit1 : Buffer  N=16
  Frame Conversion1 : FrameConversion
  Reshape3 : Reshape  OutputDimensionality=Customize  OutputDimensions=[320,1]
  Transpose1 : dspmtrx3/Transpose  Hermitian=off  overflowFlag=off
  Out1 : Outport
  wires:
  Buffer 48bit1/1 -> Transpose1/1
  Transpose1/1 -> Reshape3/1
  Reshape3/1 -> Frame Conversion1/1
  In1/1 -> Buffer 48bit1/1
  Frame Conversion1/1 -> Out1/1

== system uwb_hw_cosim_kintex/Subsystem2/Transmit2/Spreading/Hop4/Subsystem3 ==
  In1 : Inport
  Add1 : Sum  Inputs=+-
  Bi2De2 : commutil2/Bit to Integer Converter  nbits=2  bitOrder=MSB first  signedOutputValues=Unsigned  outDtype=int8  outDtypeSigned=Inherit via internal rule
  Gain2 : Gain  Gain=0.5  OutDataTypeStr=int8  RndMeth=Zero
  Gain4 : Gain  Gain=2  OutDataTypeStr=int8
  position : Outport
  sign : Outport  Port=2
  wires:
  In1/1 -> Bi2De2/1
  Gain2/1 -> Gain4/1, sign/1
  Gain4/1 -> Add1/2
  Bi2De2/1 -> Add1/1, Gain2/1
  Add1/1 -> position/1

== system uwb_hw_cosim_kintex/Subsystem2/Transmit2/Spreading/Hop4/Subsystem5 ==
  In1 : Inport
  matrix : Inport  Port=2
  CONST3 : Constant  Value=zeros(1,320)  VectorParams1D=off  OutDataTypeStr=int8  SampleTime=1
      settings: SamplingMode=Frame based
  Compare To Zero : simulink/Logic and Bit Operations/Compare To Zero  relop=>  OutDataTypeStr=uint8  ZeroCross=off
  Enabled Subsystem : Subsystem  TreatAsAtomicUnit=on
  Enabled Subsystem1 : Subsystem  TreatAsAtomicUnit=on
  Logical Operator : Logic  Operator=NOT  AllPortsSameDT=off  OutDataTypeStr=boolean
  Merge : Merge
  Reshape2 : Reshape  OutputDimensionality=Column vector (2-D)  OutputDimensions=[10,1]
  Out1 : Outport
  wires:
  CONST3/1 -> Reshape2/1
  Logical Operator/1 -> Enabled Subsystem/Enable
  Enabled Subsystem/1(Out1) -> Merge/2
  Enabled Subsystem1/1(Out1) -> Merge/1
  Compare To Zero/1 -> Enabled Subsystem1/Enable, Logical Operator/1
  Reshape2/1 -> Enabled Subsystem1/1(In1)
  matrix/1 -> Enabled Subsystem/1(In1)
  In1/1 -> Compare To Zero/1
  Merge/1 -> Out1/1

== system uwb_hw_cosim_kintex/Subsystem2/Transmit2/Spreading/Hop5/Kron ==
  p : Inport
  -p : Inport  Port=2
  sel : Inport  Port=3
  Compare To Zero : simulink/Logic and Bit Operations/Compare To Zero  relop=>  OutDataTypeStr=uint8  ZeroCross=off
  Enabled Subsystem : Subsystem  TreatAsAtomicUnit=on
  Enabled Subsystem1 : Subsystem  TreatAsAtomicUnit=on
  Logical Operator : Logic  Operator=NOT  AllPortsSameDT=off  OutDataTypeStr=boolean
  Merge : Merge
  burst : Outport
  wires:
  Logical Operator/1 -> Enabled Subsystem/Enable
  Compare To Zero/1 -> Enabled Subsystem1/Enable, Logical Operator/1
  sel/1 -> Compare To Zero/1
  -p/1 -> Enabled Subsystem/1(In1)
  Enabled Subsystem/1(Out1) -> Merge/2
  Enabled Subsystem1/1(Out1) -> Merge/1
  p/1 -> Enabled Subsystem1/1(In1)
  Merge/1 -> burst/1

== system uwb_hw_cosim_kintex/Subsystem2/Transmit2/Spreading/Hop5/Kron1 ==
  p : Inport
  -p : Inport  Port=2
  sel : Inport  Port=3
  Compare To Zero : simulink/Logic and Bit Operations/Compare To Zero  relop=>  OutDataTypeStr=uint8  ZeroCross=off
  Enabled Subsystem : Subsystem  TreatAsAtomicUnit=on
  Enabled Subsystem1 : Subsystem  TreatAsAtomicUnit=on
  Logical Operator : Logic  Operator=NOT  AllPortsSameDT=off  OutDataTypeStr=boolean
  Merge : Merge
  burst : Outport
  wires:
  Merge/1 -> burst/1
  p/1 -> Enabled Subsystem1/1(In1)
  Enabled Subsystem1/1(Out1) -> Merge/1
  Enabled Subsystem/1(Out1) -> Merge/2
  -p/1 -> Enabled Subsystem/1(In1)
  sel/1 -> Compare To Zero/1
  Compare To Zero/1 -> Logical Operator/1, Enabled Subsystem1/Enable
  Logical Operator/1 -> Enabled Subsystem/Enable

== system uwb_hw_cosim_kintex/Subsystem2/Transmit2/Spreading/Hop5/Subsystem2 ==
  note: 16bit cua S mã hóa 1 cum xung gause 320 diem, them 7x320 diem 0
      | de tao ra 1/2 frame chua tin hieu
  In1 : Inport
  Buffer 48bit1 : Buffer  N=16
  Frame Conversion1 : FrameConversion
  Reshape3 : Reshape  OutputDimensionality=Customize  OutputDimensions=[320,1]
  Transpose1 : dspmtrx3/Transpose  Hermitian=off  overflowFlag=off
  Out1 : Outport
  wires:
  Frame Conversion1/1 -> Out1/1
  In1/1 -> Buffer 48bit1/1
  Reshape3/1 -> Frame Conversion1/1
  Transpose1/1 -> Reshape3/1
  Buffer 48bit1/1 -> Transpose1/1

== system uwb_hw_cosim_kintex/Subsystem2/Transmit2/Spreading/Hop5/Subsystem3 ==
  In1 : Inport
  Add1 : Sum  Inputs=+-
  Bi2De2 : commutil2/Bit to Integer Converter  nbits=2  bitOrder=MSB first  signedOutputValues=Unsigned  outDtype=int8  outDtypeSigned=Inherit via internal rule
  Gain2 : Gain  Gain=0.5  OutDataTypeStr=int8  RndMeth=Zero
  Gain4 : Gain  Gain=2  OutDataTypeStr=int8
  position : Outport
  sign : Outport  Port=2
  wires:
  Add1/1 -> position/1
  Bi2De2/1 -> Gain2/1, Add1/1
  Gain4/1 -> Add1/2
  Gain2/1 -> sign/1, Gain4/1
  In1/1 -> Bi2De2/1

== system uwb_hw_cosim_kintex/Subsystem2/Transmit2/Spreading/Hop5/Subsystem5 ==
  In1 : Inport
  matrix : Inport  Port=2
  CONST3 : Constant  Value=zeros(1,320)  VectorParams1D=off  OutDataTypeStr=int8  SampleTime=1
      settings: SamplingMode=Frame based
  Compare To Zero : simulink/Logic and Bit Operations/Compare To Zero  relop===  OutDataTypeStr=uint8  ZeroCross=off
  Enabled Subsystem : Subsystem  TreatAsAtomicUnit=on
  Enabled Subsystem1 : Subsystem  TreatAsAtomicUnit=on
  Logical Operator : Logic  Operator=NOT  AllPortsSameDT=off  OutDataTypeStr=boolean
  Merge : Merge
  Reshape2 : Reshape  OutputDimensionality=Column vector (2-D)  OutputDimensions=[10,1]
  Out1 : Outport
  wires:
  Merge/1 -> Out1/1
  In1/1 -> Compare To Zero/1
  Reshape2/1 -> Enabled Subsystem1/1(In1)
  Compare To Zero/1 -> Logical Operator/1, Enabled Subsystem1/Enable
  Enabled Subsystem1/1(Out1) -> Merge/1
  Enabled Subsystem/1(Out1) -> Merge/2
  Logical Operator/1 -> Enabled Subsystem/Enable
  CONST3/1 -> Reshape2/1
  matrix/1 -> Enabled Subsystem/1(In1)

== system uwb_hw_cosim_kintex/Subsystem2/Transmit2/Spreading/Hop6/Kron ==
  p : Inport
  -p : Inport  Port=2
  sel : Inport  Port=3
  Compare To Zero : simulink/Logic and Bit Operations/Compare To Zero  relop=>  OutDataTypeStr=uint8  ZeroCross=off
  Enabled Subsystem : Subsystem  TreatAsAtomicUnit=on
  Enabled Subsystem1 : Subsystem  TreatAsAtomicUnit=on
  Logical Operator : Logic  Operator=NOT  AllPortsSameDT=off  OutDataTypeStr=boolean
  Merge : Merge
  burst : Outport
  wires:
  Merge/1 -> burst/1
  p/1 -> Enabled Subsystem1/1(In1)
  Enabled Subsystem1/1(Out1) -> Merge/1
  Enabled Subsystem/1(Out1) -> Merge/2
  -p/1 -> Enabled Subsystem/1(In1)
  sel/1 -> Compare To Zero/1
  Compare To Zero/1 -> Logical Operator/1, Enabled Subsystem1/Enable
  Logical Operator/1 -> Enabled Subsystem/Enable

== system uwb_hw_cosim_kintex/Subsystem2/Transmit2/Spreading/Hop6/Kron1 ==
  p : Inport
  -p : Inport  Port=2
  sel : Inport  Port=3
  Compare To Zero : simulink/Logic and Bit Operations/Compare To Zero  relop=>  OutDataTypeStr=uint8  ZeroCross=off
  Enabled Subsystem : Subsystem  TreatAsAtomicUnit=on
  Enabled Subsystem1 : Subsystem  TreatAsAtomicUnit=on
  Logical Operator : Logic  Operator=NOT  AllPortsSameDT=off  OutDataTypeStr=boolean
  Merge : Merge
  burst : Outport
  wires:
  Logical Operator/1 -> Enabled Subsystem/Enable
  Compare To Zero/1 -> Enabled Subsystem1/Enable, Logical Operator/1
  sel/1 -> Compare To Zero/1
  -p/1 -> Enabled Subsystem/1(In1)
  Enabled Subsystem/1(Out1) -> Merge/2
  Enabled Subsystem1/1(Out1) -> Merge/1
  p/1 -> Enabled Subsystem1/1(In1)
  Merge/1 -> burst/1

== system uwb_hw_cosim_kintex/Subsystem2/Transmit2/Spreading/Hop6/Subsystem2 ==
  note: 16bit cua S mã hóa 1 cum xung gause 320 diem, them 7x320 diem 0
      | de tao ra 1/2 frame chua tin hieu
  In1 : Inport
  Buffer 48bit1 : Buffer  N=16
  Frame Conversion1 : FrameConversion
  Reshape3 : Reshape  OutputDimensionality=Customize  OutputDimensions=[320,1]
  Transpose1 : dspmtrx3/Transpose  Hermitian=off  overflowFlag=off
  Out1 : Outport
  wires:
  Buffer 48bit1/1 -> Transpose1/1
  Transpose1/1 -> Reshape3/1
  Reshape3/1 -> Frame Conversion1/1
  In1/1 -> Buffer 48bit1/1
  Frame Conversion1/1 -> Out1/1

== system uwb_hw_cosim_kintex/Subsystem2/Transmit2/Spreading/Hop6/Subsystem3 ==
  In1 : Inport
  Add1 : Sum  Inputs=+-
  Bi2De2 : commutil2/Bit to Integer Converter  nbits=2  bitOrder=MSB first  signedOutputValues=Unsigned  outDtype=int8  outDtypeSigned=Inherit via internal rule
  Gain2 : Gain  Gain=0.5  OutDataTypeStr=int8  RndMeth=Zero
  Gain4 : Gain  Gain=2  OutDataTypeStr=int8
  position : Outport
  sign : Outport  Port=2
  wires:
  In1/1 -> Bi2De2/1
  Gain2/1 -> Gain4/1, sign/1
  Gain4/1 -> Add1/2
  Bi2De2/1 -> Add1/1, Gain2/1
  Add1/1 -> position/1

== system uwb_hw_cosim_kintex/Subsystem2/Transmit2/Spreading/Hop6/Subsystem5 ==
  In1 : Inport
  matrix : Inport  Port=2
  CONST3 : Constant  Value=zeros(1,320)  VectorParams1D=off  OutDataTypeStr=int8  SampleTime=1
      settings: SamplingMode=Frame based
  Compare To Zero : simulink/Logic and Bit Operations/Compare To Zero  relop===  OutDataTypeStr=uint8  ZeroCross=off
  Enabled Subsystem : Subsystem  TreatAsAtomicUnit=on
  Enabled Subsystem1 : Subsystem  TreatAsAtomicUnit=on
  Logical Operator : Logic  Operator=NOT  AllPortsSameDT=off  OutDataTypeStr=boolean
  Merge : Merge
  Reshape2 : Reshape  OutputDimensionality=Column vector (2-D)  OutputDimensions=[10,1]
  Out1 : Outport
  wires:
  matrix/1 -> Enabled Subsystem/1(In1)
  CONST3/1 -> Reshape2/1
  Logical Operator/1 -> Enabled Subsystem/Enable
  Enabled Subsystem/1(Out1) -> Merge/2
  Enabled Subsystem1/1(Out1) -> Merge/1
  Compare To Zero/1 -> Enabled Subsystem1/Enable, Logical Operator/1
  Reshape2/1 -> Enabled Subsystem1/1(In1)
  In1/1 -> Compare To Zero/1
  Merge/1 -> Out1/1

== system uwb_hw_cosim_kintex/Subsystem2/Transmit2/Spreading/Hop7/Kron ==
  p : Inport
  -p : Inport  Port=2
  sel : Inport  Port=3
  Compare To Zero : simulink/Logic and Bit Operations/Compare To Zero  relop=>  OutDataTypeStr=uint8  ZeroCross=off
  Enabled Subsystem : Subsystem  TreatAsAtomicUnit=on
  Enabled Subsystem1 : Subsystem  TreatAsAtomicUnit=on
  Logical Operator : Logic  Operator=NOT  AllPortsSameDT=off  OutDataTypeStr=boolean
  Merge : Merge
  burst : Outport
  wires:
  Logical Operator/1 -> Enabled Subsystem/Enable
  Compare To Zero/1 -> Enabled Subsystem1/Enable, Logical Operator/1
  sel/1 -> Compare To Zero/1
  -p/1 -> Enabled Subsystem/1(In1)
  Enabled Subsystem/1(Out1) -> Merge/2
  Enabled Subsystem1/1(Out1) -> Merge/1
  p/1 -> Enabled Subsystem1/1(In1)
  Merge/1 -> burst/1

== system uwb_hw_cosim_kintex/Subsystem2/Transmit2/Spreading/Hop7/Kron1 ==
  p : Inport
  -p : Inport  Port=2
  sel : Inport  Port=3
  Compare To Zero : simulink/Logic and Bit Operations/Compare To Zero  relop=>  OutDataTypeStr=uint8  ZeroCross=off
  Enabled Subsystem : Subsystem  TreatAsAtomicUnit=on
  Enabled Subsystem1 : Subsystem  TreatAsAtomicUnit=on
  Logical Operator : Logic  Operator=NOT  AllPortsSameDT=off  OutDataTypeStr=boolean
  Merge : Merge
  burst : Outport
  wires:
  Merge/1 -> burst/1
  p/1 -> Enabled Subsystem1/1(In1)
  Enabled Subsystem1/1(Out1) -> Merge/1
  Enabled Subsystem/1(Out1) -> Merge/2
  -p/1 -> Enabled Subsystem/1(In1)
  sel/1 -> Compare To Zero/1
  Compare To Zero/1 -> Logical Operator/1, Enabled Subsystem1/Enable
  Logical Operator/1 -> Enabled Subsystem/Enable

== system uwb_hw_cosim_kintex/Subsystem2/Transmit2/Spreading/Hop7/Subsystem2 ==
  note: 16bit cua S mã hóa 1 cum xung gause 320 diem, them 7x320 diem 0
      | de tao ra 1/2 frame chua tin hieu
  In1 : Inport
  Buffer 48bit1 : Buffer  N=16
  Frame Conversion1 : FrameConversion
  Reshape3 : Reshape  OutputDimensionality=Customize  OutputDimensions=[320,1]
  Transpose1 : dspmtrx3/Transpose  Hermitian=off  overflowFlag=off
  Out1 : Outport
  wires:
  Frame Conversion1/1 -> Out1/1
  In1/1 -> Buffer 48bit1/1
  Reshape3/1 -> Frame Conversion1/1
  Transpose1/1 -> Reshape3/1
  Buffer 48bit1/1 -> Transpose1/1

== system uwb_hw_cosim_kintex/Subsystem2/Transmit2/Spreading/Hop7/Subsystem3 ==
  In1 : Inport
  Add1 : Sum  Inputs=+-
  Bi2De2 : commutil2/Bit to Integer Converter  nbits=2  bitOrder=MSB first  signedOutputValues=Unsigned  outDtype=int8  outDtypeSigned=Inherit via internal rule
  Gain2 : Gain  Gain=0.5  OutDataTypeStr=int8  RndMeth=Zero
  Gain4 : Gain  Gain=2  OutDataTypeStr=int8
  position : Outport
  sign : Outport  Port=2
  wires:
  Add1/1 -> position/1
  Bi2De2/1 -> Gain2/1, Add1/1
  Gain4/1 -> Add1/2
  Gain2/1 -> sign/1, Gain4/1
  In1/1 -> Bi2De2/1

== system uwb_hw_cosim_kintex/Subsystem2/Transmit2/Spreading/Hop7/Subsystem5 ==
  In1 : Inport
  matrix : Inport  Port=2
  CONST3 : Constant  Value=zeros(1,320)  VectorParams1D=off  OutDataTypeStr=int8  SampleTime=1
      settings: SamplingMode=Frame based
  Compare To Zero : simulink/Logic and Bit Operations/Compare To Zero  relop===  OutDataTypeStr=uint8  ZeroCross=off
  Enabled Subsystem : Subsystem  TreatAsAtomicUnit=on
  Enabled Subsystem1 : Subsystem  TreatAsAtomicUnit=on
  Logical Operator : Logic  Operator=NOT  AllPortsSameDT=off  OutDataTypeStr=boolean
  Merge : Merge
  Reshape2 : Reshape  OutputDimensionality=Column vector (2-D)  OutputDimensions=[10,1]
  Out1 : Outport
  wires:
  Merge/1 -> Out1/1
  In1/1 -> Compare To Zero/1
  Reshape2/1 -> Enabled Subsystem1/1(In1)
  Compare To Zero/1 -> Logical Operator/1, Enabled Subsystem1/Enable
  Enabled Subsystem1/1(Out1) -> Merge/1
  Enabled Subsystem/1(Out1) -> Merge/2
  Logical Operator/1 -> Enabled Subsystem/Enable
  CONST3/1 -> Reshape2/1
  matrix/1 -> Enabled Subsystem/1(In1)

== system uwb_hw_cosim_kintex/Subsystem2/Transmit2/Spreading/Hop8/Kron ==
  p : Inport
  -p : Inport  Port=2
  sel : Inport  Port=3
  Compare To Zero : simulink/Logic and Bit Operations/Compare To Zero  relop=>  OutDataTypeStr=uint8  ZeroCross=off
  Enabled Subsystem : Subsystem  TreatAsAtomicUnit=on
  Enabled Subsystem1 : Subsystem  TreatAsAtomicUnit=on
  Logical Operator : Logic  Operator=NOT  AllPortsSameDT=off  OutDataTypeStr=boolean
  Merge : Merge
  burst : Outport
  wires:
  Merge/1 -> burst/1
  p/1 -> Enabled Subsystem1/1(In1)
  Enabled Subsystem1/1(Out1) -> Merge/1
  Enabled Subsystem/1(Out1) -> Merge/2
  -p/1 -> Enabled Subsystem/1(In1)
  sel/1 -> Compare To Zero/1
  Compare To Zero/1 -> Logical Operator/1, Enabled Subsystem1/Enable
  Logical Operator/1 -> Enabled Subsystem/Enable

== system uwb_hw_cosim_kintex/Subsystem2/Transmit2/Spreading/Hop8/Kron1 ==
  p : Inport
  -p : Inport  Port=2
  sel : Inport  Port=3
  Compare To Zero : simulink/Logic and Bit Operations/Compare To Zero  relop=>  OutDataTypeStr=uint8  ZeroCross=off
  Enabled Subsystem : Subsystem  TreatAsAtomicUnit=on
  Enabled Subsystem1 : Subsystem  TreatAsAtomicUnit=on
  Logical Operator : Logic  Operator=NOT  AllPortsSameDT=off  OutDataTypeStr=boolean
  Merge : Merge
  burst : Outport
  wires:
  Logical Operator/1 -> Enabled Subsystem/Enable
  Compare To Zero/1 -> Enabled Subsystem1/Enable, Logical Operator/1
  sel/1 -> Compare To Zero/1
  -p/1 -> Enabled Subsystem/1(In1)
  Enabled Subsystem/1(Out1) -> Merge/2
  Enabled Subsystem1/1(Out1) -> Merge/1
  p/1 -> Enabled Subsystem1/1(In1)
  Merge/1 -> burst/1

== system uwb_hw_cosim_kintex/Subsystem2/Transmit2/Spreading/Hop8/Subsystem2 ==
  note: 16bit cua S mã hóa 1 cum xung gause 320 diem, them 7x320 diem 0
      | de tao ra 1/2 frame chua tin hieu
  In1 : Inport
  Buffer 48bit1 : Buffer  N=16
  Frame Conversion1 : FrameConversion
  Reshape3 : Reshape  OutputDimensionality=Customize  OutputDimensions=[320,1]
  Transpose1 : dspmtrx3/Transpose  Hermitian=off  overflowFlag=off
  Out1 : Outport
  wires:
  Buffer 48bit1/1 -> Transpose1/1
  Transpose1/1 -> Reshape3/1
  Reshape3/1 -> Frame Conversion1/1
  In1/1 -> Buffer 48bit1/1
  Frame Conversion1/1 -> Out1/1
